simulink model "hf_system_fig"  (R2023b)
settings: Solver=VariableStepAuto  StartTime=0.0  StopTime=10.0  RelTol=1e-3
values from neighbouring files (symbols this model uses):
  b_adrc = 20000    [buck_control.m]
  C = 47e-6    (= 4.7e-05)    [buck_control.m]
  f = (0:Nfft/2) / Nfft    [Window.m]    (also in buck_control.m = 100000)
  L = (UI-UO)*D/(f*deta_I)    (= 8e-05)    [buck_control.m]
  R = UO / I    (= 4)    [buck_control.m]
  wc_adrc = 3000    [buck_control.m]
  wo_adrc = 5000    [buck_control.m]
undefined symbols (not defined in the file or in its folder): DiscIntNeverNeededParam
libraries: spsSeriesRLCBranchLib x11, spsCurrentMeasurementLib x4, spsGroundLib x3, spsMosfetLib x3, spsVoltageMeasurementLib x3, slpidlib x2, simulink x2, spsDCVoltageSourceLib x1, spsDiodeLib x1, spsMultiWindingTransformerLib x1, spsPowerLib x1, spsVariableResistorLib x1
settings Model: Creator=ASUS  LastModifiedBy=ASUS

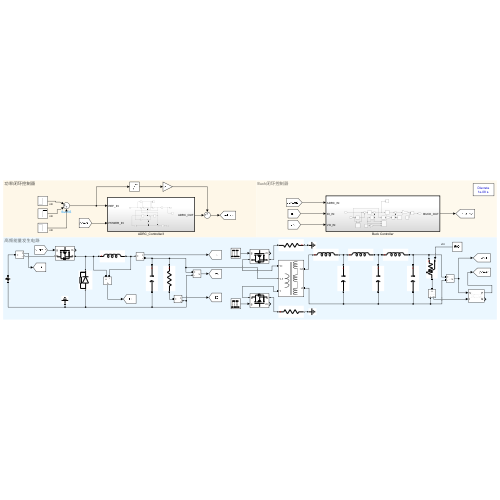
[thumbnail: Simulink's stored preview of the top-level diagram]
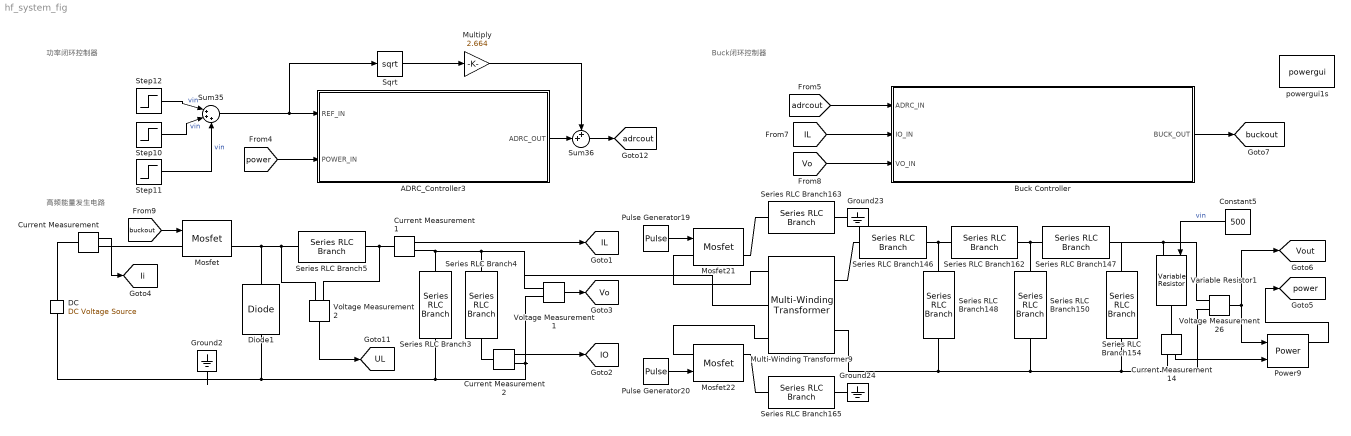
== system hf_system_fig ==
  note: 高频能量发生电路
  note: Buck闭环控制器
  note: 功率闭环控制器
  ADRC_Controller3 : Subsystem  TreatAsAtomicUnit=on  SystemSampleTime=5e-5
  Buck Controller : Subsystem  TreatAsAtomicUnit=on
  Constant5 : Constant  Value=500
  Current Measurement{,1..2,14} (4 alike) : spsCurrentMeasurementLib/Current Measurement  PhasorSimulation=off  OutputType=Complex  PSBequivalent=0
  DC : spsDCVoltageSourceLib/DC Voltage Source  Amplitude=50  Measurements=None
  Diode1 : spsDiodeLib/Diode  Ron=0.001  Lon=0  Vf=0.8  IC=0  UseSnubber=off  Rs=500  Cs=250e-9  Measurements=off
  Ground2 : spsGroundLib/Ground  LConnTagsString=a
  Ground23 : spsGroundLib/Ground  LConnTagsString=a
  Ground24 : spsGroundLib/Ground  LConnTagsString=a
  Mosfet : spsMosfetLib/Mosfet  Ron=0.1  Lon=0  Rd=0.01  Vfd=0  IC=0  Rs=1e5  Cs=inf  Measurements=on
  Mosfet21 : spsMosfetLib/Mosfet  Ron=0.1  Lon=0  Rd=0.01  Vfd=0  IC=0  Rs=1e5  Cs=inf  Measurements=on
  Mosfet22 : spsMosfetLib/Mosfet  Ron=0.1  Lon=0  Rd=0.01  Vfd=0  IC=0  Rs=1e5  Cs=inf  Measurements=on
  Multi-Winding Transformer9 : spsMultiWindingTransformerLib/Multi-Winding Transformer  LeftWindings=1  RightWindings=1  TappedWindings=taps on upper left winding  NumberOfTaps=1  SetSaturation=off  Hysteresis=off  DataFile='hysteresis.mat'  Measurements=None  UNITS=SI  NominalPower=[120 400000]  NominalVoltages=[2 4]  WindingResistances=[0 0]  WindingInductances=[0 0]  Rm=inf  Lm=inf  Saturation=[0 0;2.8284e-05 0.0097234;0.011785 0.012316]  SpecifyInitialFlux=off  InitialFlux=0  BreakLoop=off  DiscreteSolver=Trapezoidal iterative  DataType=on  TransfoNumber=1
      settings: LibrarySourceBlock=|
      | sps_lib/Power Grid Elements/Multi-Winding
      | Transformer
  Multiply : Gain  Gain=2.664
  Power9 : spsPowerLib/Power  Freq=350000  Vinit=[1, 0]  Iinit=[1, 0]  Ts=1e-8
  Pulse Generator19 : DiscretePulseGenerator  Amplitude=12  Period=286  PulseWidth=133  SampleTime=1e-8
  Pulse Generator20 : DiscretePulseGenerator  Amplitude=12  Period=286  PulseWidth=133  PhaseDelay=143  SampleTime=1e-8
  Series RLC Branch146 : spsSeriesRLCBranchLib/Series RLC Branch  LConnTagsString=__new0  RConnTagsString=__new0  BranchType=L  Resistance=1  Inductance=150e-6  SetiL0=off  InitialCurrent=0  Capacitance=1e-6  Setx0=off  InitialVoltage=0  Measurements=None
  Series RLC Branch147 : spsSeriesRLCBranchLib/Series RLC Branch  LConnTagsString=__new0  RConnTagsString=__new0  BranchType=L  Resistance=1  Inductance=150e-6  SetiL0=off  InitialCurrent=0  Capacitance=1e-6  Setx0=off  InitialVoltage=0  Measurements=None
  Series RLC Branch148 : spsSeriesRLCBranchLib/Series RLC Branch  LConnTagsString=__new0  RConnTagsString=__new0  BranchType=C  Resistance=1  Inductance=220e-6  SetiL0=off  InitialCurrent=0  Capacitance=1.451e-9  Setx0=off  InitialVoltage=0  Measurements=None
  Series RLC Branch150 : spsSeriesRLCBranchLib/Series RLC Branch  LConnTagsString=__new0  RConnTagsString=__new0  BranchType=C  Resistance=1  Inductance=220e-6  SetiL0=off  InitialCurrent=0  Capacitance=180e-12  Setx0=off  InitialVoltage=0  Measurements=None
  Series RLC Branch154 : spsSeriesRLCBranchLib/Series RLC Branch  LConnTagsString=__new0  RConnTagsString=__new0  BranchType=C  Resistance=1  Inductance=220e-6  SetiL0=off  InitialCurrent=0  Capacitance=51e-12  Setx0=off  InitialVoltage=0  Measurements=None
  Series RLC Branch162 : spsSeriesRLCBranchLib/Series RLC Branch  LConnTagsString=__new0  RConnTagsString=__new0  BranchType=L  Resistance=1  Inductance=220e-6  SetiL0=off  InitialCurrent=0  Capacitance=1e-6  Setx0=off  InitialVoltage=0  Measurements=None
  Series RLC Branch163 : spsSeriesRLCBranchLib/Series RLC Branch  LConnTagsString=__new0  RConnTagsString=__new0  BranchType=R  Resistance=0.02  Inductance=220e-6  SetiL0=off  InitialCurrent=0  Capacitance=180e-12  Setx0=off  InitialVoltage=0  Measurements=None
  Series RLC Branch165 : spsSeriesRLCBranchLib/Series RLC Branch  LConnTagsString=__new0  RConnTagsString=__new0  BranchType=R  Resistance=0.02  Inductance=220e-6  SetiL0=off  InitialCurrent=0  Capacitance=180e-12  Setx0=off  InitialVoltage=0  Measurements=None
  Series RLC Branch3 : spsSeriesRLCBranchLib/Series RLC Branch  LConnTagsString=__new0  RConnTagsString=__new0  BranchType=C  Resistance=1  Inductance=0.6e-3  SetiL0=off  InitialCurrent=0  Capacitance=C  Setx0=off  InitialVoltage=100  Measurements=None
  Series RLC Branch4 : spsSeriesRLCBranchLib/Series RLC Branch  LConnTagsString=__new0  RConnTagsString=__new0  BranchType=R  Resistance=R  Inductance=0.6e-3  SetiL0=off  InitialCurrent=0  Capacitance=C  Setx0=off  InitialVoltage=100  Measurements=None
  Series RLC Branch5 : spsSeriesRLCBranchLib/Series RLC Branch  LConnTagsString=__new0  RConnTagsString=__new0  BranchType=L  Resistance=1  Inductance=L  SetiL0=off  InitialCurrent=0  Capacitance=1e-6  Setx0=off  InitialVoltage=0  Measurements=None
  Sqrt : Sqrt
  Step10 : Step  Time=0.02  After=20  SampleTime=5e-5
  Step11 : Step  Time=0.04  After=-20  SampleTime=5e-5
  Step12 : Step  Time=0  After=20  SampleTime=5e-5
  Sum35 : Sum  Inputs=|+++
  Sum36 : Sum  Inputs=++|
  Variable Resistor1 : spsVariableResistorLib/Variable Resistor  Rabsmin=0
      settings: LibrarySourceBlock=sps_lib/Passives/Variable Resistor
  Voltage Measurement1 : spsVoltageMeasurementLib/Voltage Measurement  PhasorSimulation=off  OutputType=Complex  PSBequivalent=0
  Voltage Measurement2 : spsVoltageMeasurementLib/Voltage Measurement  PhasorSimulation=off  OutputType=Complex  PSBequivalent=0
  Voltage Measurement26 : spsVoltageMeasurementLib/Voltage Measurement  PhasorSimulation=off  OutputType=Complex  PSBequivalent=0
  powergui1s : spspowerguiLib/powergui  Priority=1  SimulationMode=Discrete  SampleTime=1e-8  frequency=60  Iterations=50  frequencyindice=0  Pbase=100e6  ErrMax=1e-4  UnitsV=kV  UnitsW=MW  buscounter=0  FunctionMessages=off  echomessages=off  EnableUseOfTLC=off  CurrentSourceSwitches=off  DisableSnubberDevices=off  DisableRonSwitches=off  DisableVfSwitches=off  DisplayEquations=off  AutomaticDiscreteSolvers=off  SolverType=Tustin/Backward Euler (TBE)  Interpol=off  ExternalGateDelay=off  methode=off  Ts=10  x0status=blocks  SPID=off  SwTol=0  HookPort=off  NonlinearTolerance=1e-4  nMaxIteration=100  ContinueOnMaxIteration=off  RestoreLinks=warning  ResistiveCurrentMeasurement=off  Frange=[0:2:500]  Ylog=off  Xlog=on  ShowGrid=off  save=off  variable=ZData  structure=0  ZoomFFT=off  StartTime=0.0  cycles=1  DisplayStyle=1  fundamental=60  FreqAxis=off  MaxFrequency=1000  frequencyindicesteady=1  RmsSteady=1  display=off
  tag scope: IL=global, IO=global, Ii=global, UL=global, Vo=global, Vout=global, adrcout=global, buckout=global, power=global
  wires:
  Current Measurement/1 -> [Ii]
  Voltage Measurement1/1 -> [Vo]
  Voltage Measurement2/1 -> [UL]
  Current Measurement2/1 -> [IO]
  [buckout] -> Mosfet/1
  Current Measurement1/1 -> [IL]
  Voltage Measurement26/1 -> Power9/1, [Vout]
  Current Measurement14/1 -> Power9/2
  Pulse Generator20/1 -> Mosfet22/1
  Power9/1 -> [power]
  Constant5/1 -> Variable Resistor1/1  "vin"
  Pulse Generator19/1 -> Mosfet21/1
  [IL] -> Buck Controller/2(IO_IN)
  [Vo] -> Buck Controller/3(VO_IN)
  Buck Controller/1(BUCK_OUT) -> [buckout]
  [adrcout] -> Buck Controller/1(ADRC_IN)
  Step11/1 -> Sum35/3  "vin"
  Step12/1 -> Sum35/1  "vin"
  Sqrt/1 -> Multiply/1
  Sum36/1 -> [adrcout]
  ADRC_Controller3/1(ADRC_OUT) -> Sum36/2
  Sum35/1 -> Sqrt/1, ADRC_Controller3/1(REF_IN)
  Step10/1 -> Sum35/2  "vin"
  Multiply/1 -> Sum36/1
  [power] -> ADRC_Controller3/2(POWER_IN)
  connections:
  Voltage Measurement1/LConn2 -- Current Measurement2/RConn1 -- Series RLC Branch3/RConn1 -- Ground2/LConn1 -- DC/LConn1 -- Diode1/LConn1
  Voltage Measurement2/LConn2 -- Series RLC Branch5/RConn1 -- Current Measurement1/LConn1
  Series RLC Branch4/LConn1 -- Voltage Measurement1/LConn1 -- Multi-Winding Transformer9/LConn2 -- Series RLC Branch3/LConn1 -- Current Measurement1/RConn1
  Diode1/RConn1 -- Mosfet/RConn1 -- Voltage Measurement2/LConn1 -- Series RLC Branch5/LConn1
  Current Measurement2/LConn1 -- Series RLC Branch4/RConn1
  Mosfet/LConn1 -- Current Measurement/RConn1
  Current Measurement/LConn1 -- DC/RConn1
  Voltage Measurement26/LConn1 -- Series RLC Branch154/LConn1 -- Series RLC Branch147/RConn1 -- Variable Resistor1/LConn1
  Series RLC Branch148/RConn1 -- Multi-Winding Transformer9/RConn2 -- Series RLC Branch150/RConn1 -- Series RLC Branch154/RConn1 -- Voltage Measurement26/LConn2 -- Current Measurement14/RConn1
  Series RLC Branch162/RConn1 -- Series RLC Branch150/LConn1 -- Series RLC Branch147/LConn1
  Series RLC Branch148/LConn1 -- Series RLC Branch162/LConn1 -- Series RLC Branch146/RConn1
  Mosfet22/LConn1 -- Multi-Winding Transformer9/LConn3
  Series RLC Branch165/LConn1 -- Mosfet22/RConn1
  Mosfet21/LConn1 -- Multi-Winding Transformer9/LConn1
  Current Measurement14/LConn1 -- Variable Resistor1/RConn1
  Ground24/LConn1 -- Series RLC Branch165/RConn1
  Series RLC Branch163/RConn1 -- Mosfet21/RConn1
  Series RLC Branch163/LConn1 -- Ground23/LConn1
  Multi-Winding Transformer9/RConn1 -- Series RLC Branch146/LConn1

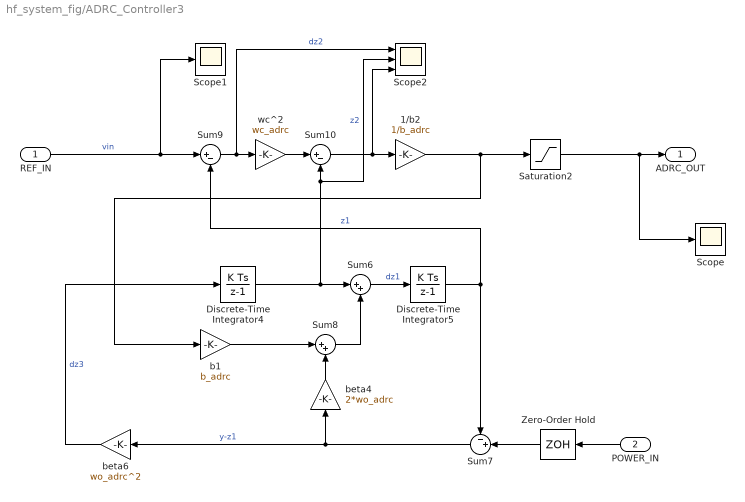
== system hf_system_fig/ADRC_Controller3 ==
  REF_IN : Inport
  POWER_IN : Inport  Port=2
  1/b2 : Gain  Gain=1/b_adrc
  Discrete-Time Integrator4 : DiscreteIntegrator  SampleTime=-1  ICPrevOutput=DiscIntNeverNeededParam  ICPrevScaledInput=DiscIntNeverNeededParam
  Discrete-Time Integrator5 : DiscreteIntegrator  SampleTime=-1  ICPrevOutput=DiscIntNeverNeededParam  ICPrevScaledInput=DiscIntNeverNeededParam
  Saturation2 : Saturate  UpperLimit=40  LowerLimit=-40
  Scope : Scope
  Scope1 : Scope
  Scope2 : Scope  NumInputPorts=3
  Sum10 : Sum  Inputs=|+-
  Sum6 : Sum  Inputs=|++
  Sum7 : Sum  Inputs=-+|
  Sum8 : Sum  Inputs=|++
  Sum9 : Sum  Inputs=|+-
  Zero-Order Hold : ZeroOrderHold  SampleTime=-1
  b1 : Gain  Gain=b_adrc
  beta4 : Gain  Gain=2*wo_adrc
  beta6 : Gain  Gain=wo_adrc^2
  wc^2 : Gain  Gain=wc_adrc
  ADRC_OUT : Outport
  wires:
  Sum7/1 -> beta4/1, beta6/1  "y-z1"
  1/b2/1 -> Saturation2/1, b1/1
  wc^2/1 -> Sum10/1
  Sum9/1 -> Scope2/1, wc^2/1  "dz2"
  REF_IN/1 -> Scope1/1, Sum9/1  "vin"
  beta6/1 -> Discrete-Time Integrator4/1  "dz3"
  POWER_IN/1 -> Zero-Order Hold/1
  Sum6/1 -> Discrete-Time Integrator5/1  "dz1"
  Discrete-Time Integrator5/1 -> Sum7/1, Sum9/2  "z1"
  b1/1 -> Sum8/1
  Discrete-Time Integrator4/1 -> Scope2/2, Sum10/2, Sum6/1  "z2"
  Zero-Order Hold/1 -> Sum7/2
  beta4/1 -> Sum8/2
  Sum8/1 -> Sum6/2
  Sum10/1 -> Scope2/3, 1/b2/1
  Saturation2/1 -> Scope/1, ADRC_OUT/1

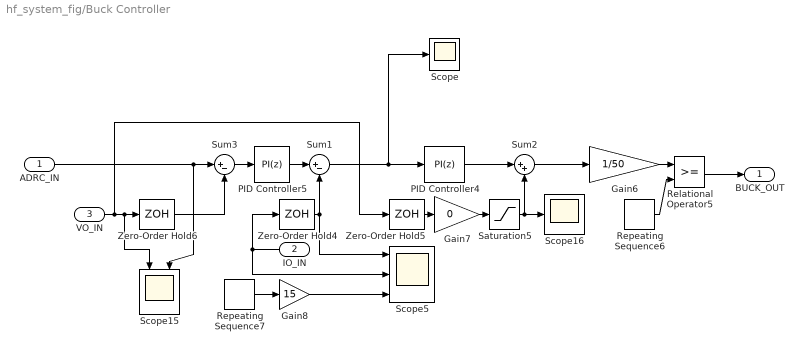
== system hf_system_fig/Buck Controller ==
  ADRC_IN : Inport
  IO_IN : Inport  Port=2
  VO_IN : Inport  Port=3
  Gain6 : Gain  Gain=1/50
  Gain7 : Gain  Gain=0
  Gain8 : Gain  Gain=15
  PID Controller4 : slpidlib/PID Controller  Controller=PI  Form=Parallel  TimeDomain=Discrete-time  UseExternalTs=off  SampleTime=1/f  IntegratorMethod=Trapezoidal  FilterMethod=Forward Euler  ControllerParametersSource=internal  P=10  I=50000  UseKiTs=off  D=0  N=100  UseFilter=on  TunerSelectOption=Transfer Function Based (PID Tuner App)  InitialConditionSource=internal  InitialConditionForIntegrator=0  InitialConditionForFilter=0  DifferentiatorICPrevScaledInput=0  ExternalReset=none  TrackingMode=off  Kt=1  LimitOutput=on  SatLimitsSource=internal  UpperSaturationLimit=50  LowerSaturationLimit=-50  LinearizeAsGain=on  AntiWindupMode=none  Kb=1  LimitIntegrator=off  UpperIntegratorSaturationLimit=inf  LowerIntegratorSaturationLimit=-inf  POutMin=[]  POutMax=[]  IOutMin=[]  IOutMax=[]  DOutMin=[]  DOutMax=[]  NOutMin=[]  NOutMax=[]  SumOutMin=[]  SumOutMax=[]  SaturationOutMin=[]  SaturationOutMax=[]  PParamMin=[]  PParamMax=[]  IParamMin=[]  IParamMax=[]  DParamMin=[]  DParamMax=[]  NParamMin=[]  NParamMax=[]  KbParamMin=[]  KbParamMax=[]  KtParamMin=[]  KtParamMax=[]  KbOutMin=[]  KbOutMax=[]  KtOutMin=[]  KtOutMax=[]  IntegratorOutMin=[]  IntegratorOutMax=[]  FilterOutMin=[]  FilterOutMax=[]  SumI1OutMin=[]  SumI1OutMax=[]  SumI2OutMin=[]  SumI2OutMax=[]  SumI3OutMin=[]  SumI3OutMax=[]  SumI4OutMin=[]  SumI4OutMax=[]  SumDOutMin=[]  SumDOutMax=[]  DifferentiatorOutMin=[]  DifferentiatorOutMax=[]  FilterDiffOutCoefMin=[]  FilterDiffOutCoefMax=[]  ReciprocalOutMin=[]  ReciprocalOutMax=[]  SumDenOutMin=[]  SumDenOutMax=[]  SumNumOutMin=[]  SumNumOutMax=[]  DivideOutMin=[]  DivideOutMax=[]  UdiffTsProdOutMin=[]  UdiffTsProdOutMax=[]  NTsProdOutMin=[]  NTsProdOutMax=[]  UintegralTsProdOutMin=[]  UintegralTsProdOutMax=[]  UngainTsProdOutMin=[]  UngainTsProdOutMax=[]  ClampingZeroOutDataTypeStr=Inherit: Inherit via back propagation  ClampingZeroOutMin=[]  ClampingZeroOutMax=[]  FilterDenConstantOutDataTypeStr=Inherit: Inherit via back propagation  FilterDenConstantOutMin=[]  FilterDenConstantOutMax=[]  PCopyOutDataTypeStr=Inherit: Inherit via back propagation  PCopyOutMin=[]  PCopyOutMax=[]  NCopyOutDataTypeStr=Inherit: Inherit via back propagation  NCopyOutMin=[]  NCopyOutMax=[]  IntegratorContinuousStateAttributes=''  IntegratorStateMustResolveToSignalObject=off  IntegratorRTWStateStorageClass=Auto  FilterContinuousStateAttributes=''  FilterStateMustResolveToSignalObject=off  FilterRTWStateStorageClass=Auto  ParallelPVariant=InternalParameters  IdealPVariant=Disabled  IVariant=InternalParameters  DVariant=Disabled  IntegratorVariant=Discrete  SatVariant=Enabled  AWVariant=Passthrough  PCopyVariant=Disabled  TRVariant=Disabled  FdbkBlocksVariant=Forward  IdealPFdbkVariant=Disabled  SatFdbkVariant=Disabled  DerivativeFilterVariant=Disabled  NVariant=Disabled  NCopyVariant=Disabled_SignalSpec  FilterICVariant=Disabled  IntegratorICVariant=InternalICs  ExternalResetVariant=Disabled  TRSumVariant=Passthrough  SumFdbkVariant=Disabled  SumVariant=Sum_PI  TsampFilterVariant=InternalTs  TsampNgainVariant=Passthrough  TsampIntegralVariant=Disabled_SignalSpec  ExternalSaturationOutDataTypeStr=Inherit: Same as second input
  PID Controller5 : slpidlib/PID Controller  Controller=PI  Form=Parallel  TimeDomain=Discrete-time  UseExternalTs=off  SampleTime=1/f  IntegratorMethod=Trapezoidal  FilterMethod=Forward Euler  ControllerParametersSource=internal  P=0.8  I=1000  UseKiTs=off  D=0  N=100  UseFilter=on  TunerSelectOption=Transfer Function Based (PID Tuner App)  InitialConditionSource=internal  InitialConditionForIntegrator=0  InitialConditionForFilter=0  DifferentiatorICPrevScaledInput=0  ExternalReset=none  TrackingMode=off  Kt=1  LimitOutput=on  SatLimitsSource=internal  UpperSaturationLimit=20  LowerSaturationLimit=0  LinearizeAsGain=on  AntiWindupMode=none  Kb=1  LimitIntegrator=off  UpperIntegratorSaturationLimit=inf  LowerIntegratorSaturationLimit=-inf  POutMin=[]  POutMax=[]  IOutMin=[]  IOutMax=[]  DOutMin=[]  DOutMax=[]  NOutMin=[]  NOutMax=[]  SumOutMin=[]  SumOutMax=[]  SaturationOutMin=[]  SaturationOutMax=[]  PParamMin=[]  PParamMax=[]  IParamMin=[]  IParamMax=[]  DParamMin=[]  DParamMax=[]  NParamMin=[]  NParamMax=[]  KbParamMin=[]  KbParamMax=[]  KtParamMin=[]  KtParamMax=[]  KbOutMin=[]  KbOutMax=[]  KtOutMin=[]  KtOutMax=[]  IntegratorOutMin=[]  IntegratorOutMax=[]  FilterOutMin=[]  FilterOutMax=[]  SumI1OutMin=[]  SumI1OutMax=[]  SumI2OutMin=[]  SumI2OutMax=[]  SumI3OutMin=[]  SumI3OutMax=[]  SumI4OutMin=[]  SumI4OutMax=[]  SumDOutMin=[]  SumDOutMax=[]  DifferentiatorOutMin=[]  DifferentiatorOutMax=[]  FilterDiffOutCoefMin=[]  FilterDiffOutCoefMax=[]  ReciprocalOutMin=[]  ReciprocalOutMax=[]  SumDenOutMin=[]  SumDenOutMax=[]  SumNumOutMin=[]  SumNumOutMax=[]  DivideOutMin=[]  DivideOutMax=[]  UdiffTsProdOutMin=[]  UdiffTsProdOutMax=[]  NTsProdOutMin=[]  NTsProdOutMax=[]  UintegralTsProdOutMin=[]  UintegralTsProdOutMax=[]  UngainTsProdOutMin=[]  UngainTsProdOutMax=[]  ClampingZeroOutDataTypeStr=Inherit: Inherit via back propagation  ClampingZeroOutMin=[]  ClampingZeroOutMax=[]  FilterDenConstantOutDataTypeStr=Inherit: Inherit via back propagation  FilterDenConstantOutMin=[]  FilterDenConstantOutMax=[]  PCopyOutDataTypeStr=Inherit: Inherit via back propagation  PCopyOutMin=[]  PCopyOutMax=[]  NCopyOutDataTypeStr=Inherit: Inherit via back propagation  NCopyOutMin=[]  NCopyOutMax=[]  IntegratorContinuousStateAttributes=''  IntegratorStateMustResolveToSignalObject=off  IntegratorRTWStateStorageClass=Auto  FilterContinuousStateAttributes=''  FilterStateMustResolveToSignalObject=off  FilterRTWStateStorageClass=Auto  ParallelPVariant=InternalParameters  IdealPVariant=Disabled  IVariant=InternalParameters  DVariant=Disabled  IntegratorVariant=Discrete  SatVariant=Enabled  AWVariant=Passthrough  PCopyVariant=Disabled  TRVariant=Disabled  FdbkBlocksVariant=Forward  IdealPFdbkVariant=Disabled  SatFdbkVariant=Disabled  DerivativeFilterVariant=Disabled  NVariant=Disabled  NCopyVariant=Disabled_SignalSpec  FilterICVariant=Disabled  IntegratorICVariant=InternalICs  ExternalResetVariant=Disabled  TRSumVariant=Passthrough  SumFdbkVariant=Disabled  SumVariant=Sum_PI  TsampFilterVariant=InternalTs  TsampNgainVariant=Passthrough  TsampIntegralVariant=Disabled_SignalSpec  ExternalSaturationOutDataTypeStr=Inherit: Same as second input
  Relational Operator5 : RelationalOperator  OutDataTypeStr=boolean  RndMeth=Simplest  InputSameDT=off
  Repeating Sequence6 : simulink/Sources/Repeating Sequence  rep_seq_t=[0 1/f]  rep_seq_y=[0 1]
  Repeating Sequence7 : simulink/Sources/Repeating Sequence  rep_seq_t=[0 1/f]  rep_seq_y=[0 1]
  Saturation5 : Saturate  UpperLimit=50  LowerLimit=0
  Scope : Scope
  Scope15 : Scope  NumInputPorts=2
  Scope16 : Scope
  Scope5 : Scope  NumInputPorts=3
  Sum1 : Sum  Inputs=|+-
  Sum2 : Sum  Inputs=|++
  Sum3 : Sum  Inputs=|+-
  Zero-Order Hold4 : ZeroOrderHold  SampleTime=1/f
  Zero-Order Hold5 : ZeroOrderHold  SampleTime=1/f
  Zero-Order Hold6 : ZeroOrderHold  SampleTime=1/f
  BUCK_OUT : Outport
  wires:
  Relational Operator5/1 -> BUCK_OUT/1
  Sum1/1 -> Scope/1, PID Controller4/1
  Zero-Order Hold4/1 -> Scope5/1, Sum1/2
  Sum3/1 -> PID Controller5/1
  Gain7/1 -> Saturation5/1
  PID Controller4/1 -> Sum2/1
  ADRC_IN/1 -> Scope15/2, Sum3/1
  Gain6/1 -> Relational Operator5/1
  PID Controller5/1 -> Sum1/1
  Repeating Sequence6/1 -> Relational Operator5/2
  Sum2/1 -> Gain6/1
  VO_IN/1 -> Zero-Order Hold5/1, Scope15/1, Zero-Order Hold6/1
  Zero-Order Hold5/1 -> Gain7/1
  Zero-Order Hold6/1 -> Sum3/2
  Gain8/1 -> Scope5/3
  Saturation5/1 -> Sum2/2, Scope16/1
  Repeating Sequence7/1 -> Gain8/1
  IO_IN/1 -> Scope5/2, Zero-Order Hold4/1
